simulink subsystem "ICM_20608_G"  (R2025b)
settings: Solver=VariableStepAuto  StartTime=0.0  StopTime=10.0  RelTol=1e-3
undefined symbols (not defined in the file): ba_low_init, bg_init
settings Model: Creator=jak64  LastModifiedBy=slee7

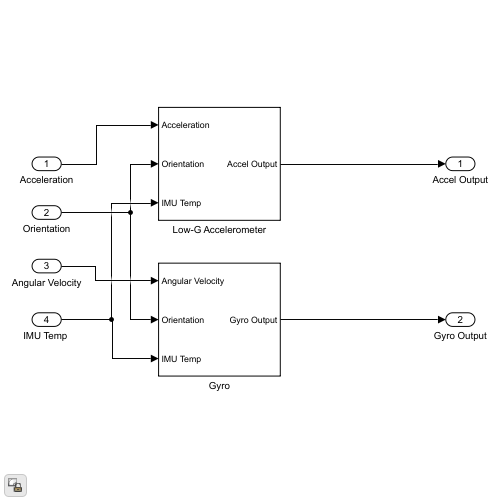
[thumbnail: Simulink's stored preview of the top-level diagram]
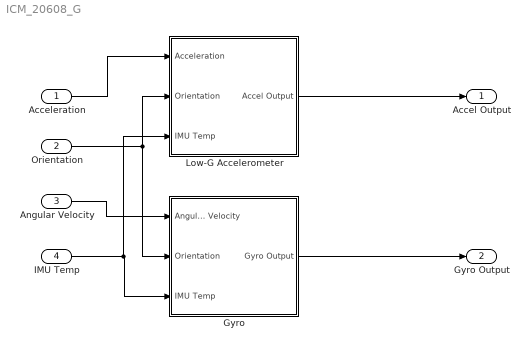
== system ICM_20608_G ==
  Acceleration : Inport
  Orientation : Inport  Port=2
  Angular Velocity : Inport  Port=3
  "IMU Temp " : Inport  Port=4
  Gyro : Subsystem
  Low-G Accelerometer : Subsystem
  Accel Output : Outport
  Gyro Output : Outport  Port=2
  wires:
  "IMU Temp "/1 -> Gyro/3(IMU Temp), Low-G Accelerometer/3(IMU Temp)
  Angular Velocity/1 -> Gyro/1(Angular Velocity)
  Orientation/1 -> Low-G Accelerometer/2(Orientation), Gyro/2(Orientation)
  Acceleration/1 -> Low-G Accelerometer/1(Acceleration)
  Low-G Accelerometer/1(Accel Output) -> Accel Output/1
  Gyro/1(Gyro Output) -> Gyro Output/1

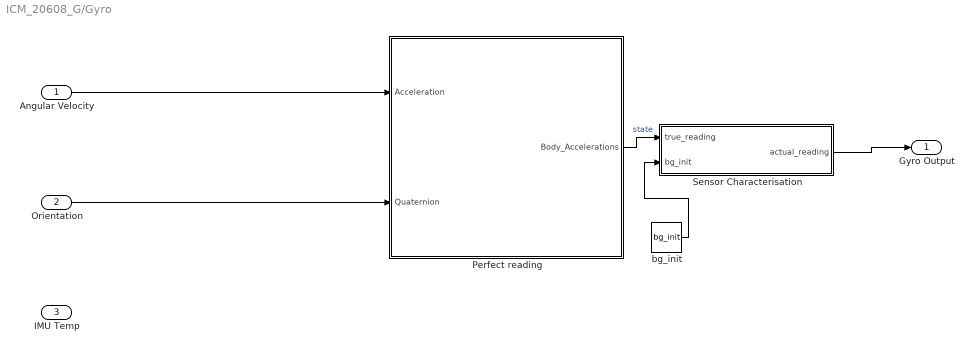
== system ICM_20608_G/Gyro ==
  Angular Velocity : Inport
  Orientation : Inport  Port=2
  IMU Temp : Inport  Port=3
  Perfect reading : MATLAB Function  TreatAsAtomicUnit=on
  Sensor Characterisation : MATLAB Function  TreatAsAtomicUnit=on
  bg_init : Constant  Value=bg_init
  Gyro Output : Outport
  wires:
  bg_init/1 -> Sensor Characterisation/2(bg_init)
  Perfect reading/1(Body_Accelerations) -> Sensor Characterisation/1(true_reading)  "state"
  Sensor Characterisation/1(actual_reading) -> Gyro Output/1
  Orientation/1 -> Perfect reading/2(Quaternion)
  Angular Velocity/1 -> Perfect reading/1(Acceleration)

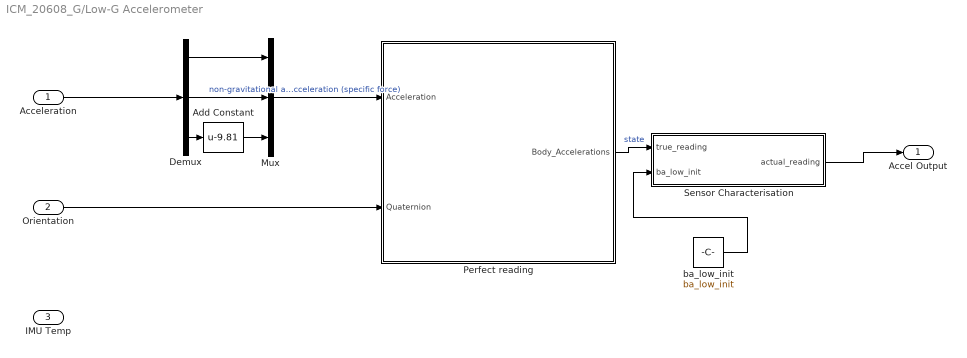
== system ICM_20608_G/Low-G Accelerometer ==
  Acceleration : Inport
  Orientation : Inport  Port=2
  IMU Temp : Inport  Port=3
  Add Constant : Bias  Bias=-9.81  SaturateOnIntegerOverflow=off
  Demux : Demux  Outputs=3
  Mux : Mux  Inputs=3
  Perfect reading : MATLAB Function  TreatAsAtomicUnit=on
  Sensor Characterisation : MATLAB Function  TreatAsAtomicUnit=on
  ba_low_init : Constant  Value=ba_low_init
  Accel Output : Outport
  wires:
  ba_low_init/1 -> Sensor Characterisation/2(ba_low_init)
  Perfect reading/1(Body_Accelerations) -> Sensor Characterisation/1(true_reading)  "state"
  Sensor Characterisation/1(actual_reading) -> Accel Output/1
  Add Constant/1 -> Mux/3
  Demux/1 -> Mux/1
  Demux/2 -> Mux/2
  Mux/1 -> Perfect reading/1(Acceleration)  "non-gravitational acceleration (specific force)"
  Demux/3 -> Add Constant/1
  Orientation/1 -> Perfect reading/2(Quaternion)
  Acceleration/1 -> Demux/1

== matlab function ICM_20608_G/Gyro/Perfect reading ==
  data: Acceleration input; Body_Accelerations output; Quaternion input
function Body_Accelerations = accel_sensor(Acceleration, Quaternion)
%#codegen
Body_Accelerations = ned2body(Acceleration, Quaternion);
end

== matlab function ICM_20608_G/Gyro/Sensor Characterisation ==
  settings: updateMethod=DISCRETE
  data: true_reading input; actual_reading output; bg_init input
function actual_reading = fcn(true_reading, bg_init)
    persistent b_previous

    dt = 0.0553; % Simulation Time Step[s]

    % Bias: Composite Bias = Const + Gauss-Markov Drift
    
        b_const = bg_init'; % Constant bias
    
        % Drift bias (b = exp^-dt/tau * b_previous + omega)
        
        if isempty(b_previous)
            b_previous = [0; 0; 0]; 
        end
    
        tau = [1.105; 1.105; 1.105]; % time constant of drift
        q = [4.390573e-05; 2.319960e-05; 1.494807e-05]; % variance on drift
    
        omega = sqrt(q) .* randn(3,1); % omega ~ N(0,q)
        
        b_drift = exp(-dt ./ tau) .* b_previous + omega;
    
        composite_bias = b_const + b_drift; 

    % Noise: Gaussian  

        noise_variance = [0.130937;  0.093580;  0.075444]; 
    
        noise = noise_variance .* randn(3,1); 
    
    % Quantisation:

        quant_step = 0.05; % Quant Step
   

    % Reading Processing:

        actual_reading_continuous  = true_reading(:) + composite_bias + noise;

        actual_reading_quantised = quant_step .* round(actual_reading_continuous ./ quant_step);

        actual_reading = actual_reading_quantised; 

end

% Currently Ignoring: 
% Scale_factor_error 
% Misalignment_error

== matlab function ICM_20608_G/Low-G Accelerometer/Perfect reading ==
  data: Acceleration input; Body_Accelerations output; Quaternion input
function Body_Accelerations = accel_sensor(Acceleration, Quaternion)
%#codegen
Body_Accelerations = ned2body(Acceleration, Quaternion);
end

== matlab function ICM_20608_G/Low-G Accelerometer/Sensor Characterisation ==
  data: true_reading input; actual_reading output; ba_low_init input
function actual_reading = fcn(true_reading, ba_low_init)
    persistent b_previous

    dt = 0.0553; % Simulation Time Step[s]

    % Bias: Composite Bias = Const + Gauss-Markov Drift
    
        b_const = ba_low_init'; % Constant bias
    
        % Drift bias (b = exp^-dt/tau * b_previous + omega)
        
        if isempty(b_previous)
            b_previous = [0; 0; 0]; 
        end
    
        tau = [1.437; 1.437; 1.437]; % time constant of drift
        q = [1.483796e-06; 1.224280e-06; 1.983171e-06]; % variance on drift
    
        omega = sqrt(q) .* randn(3,1); % omega ~ N(0,q)
        
        b_drift = exp(-dt ./ tau) .* b_previous + omega;
    
        composite_bias = b_const + b_drift; 

    % Noise: Gaussian  

        noise_variance = [0.020005; 0.021677; 0.025995]; 
    
        noise = noise_variance .* randn(3,1); 
    
    % Quantisation:

        quant_step = 0.004905; % Quant Step: data sheet
   

    % Reading Processing:

        actual_reading_continuous  = true_reading(:) + composite_bias + noise;

        actual_reading_quantised = quant_step .* round(actual_reading_continuous./quant_step);

        actual_reading = actual_reading_quantised; 

end

% Currently Ignoring: 
% Scale_factor_error 
% Misalignment_error
